simulink model "Bebop_sim_joystick_pathtrack"  (R2018a)
settings: Solver=VariableStepAuto  StartTime=0.0  StopTime=50  FixedStep=.05  MaxStep=0.3  MinStep=0.002
values from neighbouring files (symbols this model uses):
  g = 9.81    [initialize_race_no_realtime.m]    (also in initialize_race_realtime.m; initialize_race_realtime_backup_cubic.m; moving_average_rls_own.m = P(i-1)*meas*(lambda+meas*P(i-1)*meas)^-1)
  max_theta_X = (40)*pi/180    (= 0.698131700798)    [Bebop_sim_init.m]    (also in initialize_race_no_realtime.m = 0.13962634016; initialize_race_realtime.m = 1.308996939; initialize_race_realtime_backup_cubic.m = 1.308996939; run_batch1.m = list_agility(idx_agility)*max_theta_X)
  max_theta_Y = (40)*pi/180    (= 0.698131700798)    [Bebop_sim_init.m]    (also in initialize_race_no_realtime.m = 0.13962634016; initialize_race_realtime.m = 1.308996939; initialize_race_realtime_backup_cubic.m = 1.308996939; run_batch1.m = list_agility(idx_agility)*max_theta_Y)
  max_v_Z = .5    (= 0.5)    [Bebop_sim_init.m]    (also in initialize_race_no_realtime.m = 1; initialize_race_realtime.m = 3; initialize_race_realtime_backup_cubic.m = 3; run_batch1.m = list_agility(idx_agility)*max_v_Z)
libraries: simulink x2, sharedtransform x1, vrlib x1
settings Model: EnablePacing=on  Creator=vinni  LastModifiedBy=vinni
settings HardwareCC: ProdBitPerLong=64  ProdHWDeviceType=Intel->x86-64 (Linux 64)

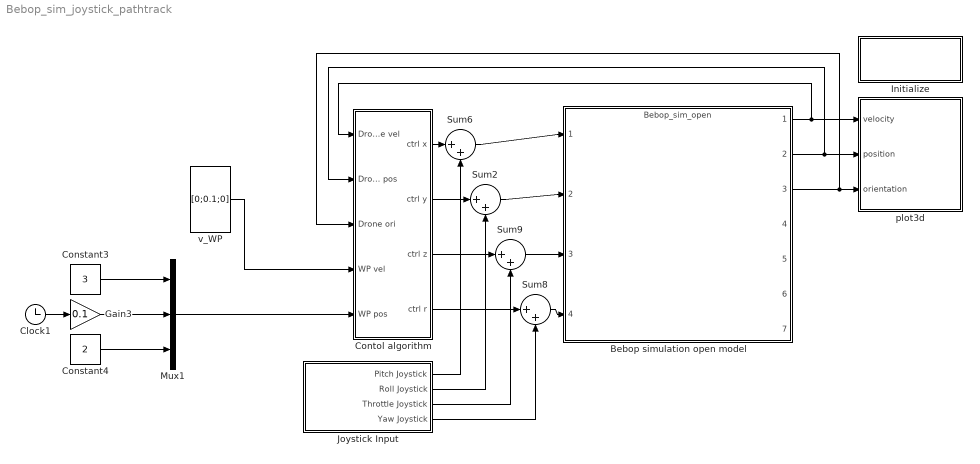
== system Bebop_sim_joystick_pathtrack ==
  Bebop simulation open model : ModelReference  ModelNameDialog=Bebop_sim_open.slx  SimulationMode=Normal  ModelReferenceVersion=1.31
  Clock1 : Clock
  Constant3 : Constant  Value=3
  Constant4 : Constant  Value=2
  Contol algorithm : Subsystem
  Gain3 : Gain  Gain=0.1
  Initialize : Subsystem  TreatAsAtomicUnit=on
  Joystick Input : Subsystem
  Mux1 : Mux  Inputs=3
  Sum{2,6,8..9} (4 alike) : Sum  Inputs=|++
  plot3d : MATLAB Function  TreatAsAtomicUnit=on
  v_WP : Constant  Value=[0;0.1;0]  VectorParams1D=off
  wires:
  Bebop simulation open model/2 -> plot3d/2(position), Contol algorithm/2(Drone pos)
  Bebop simulation open model/3 -> plot3d/3(orientation), Contol algorithm/3(Drone ori)
  Sum2/1 -> Bebop simulation open model/2
  Joystick Input/2(Roll Joystick) -> Sum2/2
  Joystick Input/1(Pitch Joystick) -> Sum6/2
  Joystick Input/4(Yaw Joystick) -> Sum8/2
  Joystick Input/3(Throttle Joystick) -> Sum9/2
  Bebop simulation open model/1 -> Contol algorithm/1(Drone vel), plot3d/1(velocity)
  Sum6/1 -> Bebop simulation open model/1
  Sum8/1 -> Bebop simulation open model/4
  Clock1/1 -> Gain3/1
  Sum9/1 -> Bebop simulation open model/3
  Gain3/1 -> Mux1/2
  Constant3/1 -> Mux1/1
  Constant4/1 -> Mux1/3
  v_WP/1 -> Contol algorithm/4(WP vel)
  Mux1/1 -> Contol algorithm/5(WP pos)
  Contol algorithm/1(ctrl x) -> Sum6/1
  Contol algorithm/2(ctrl y) -> Sum2/1
  Contol algorithm/3(ctrl z) -> Sum9/1
  Contol algorithm/4(ctrl r) -> Sum8/1

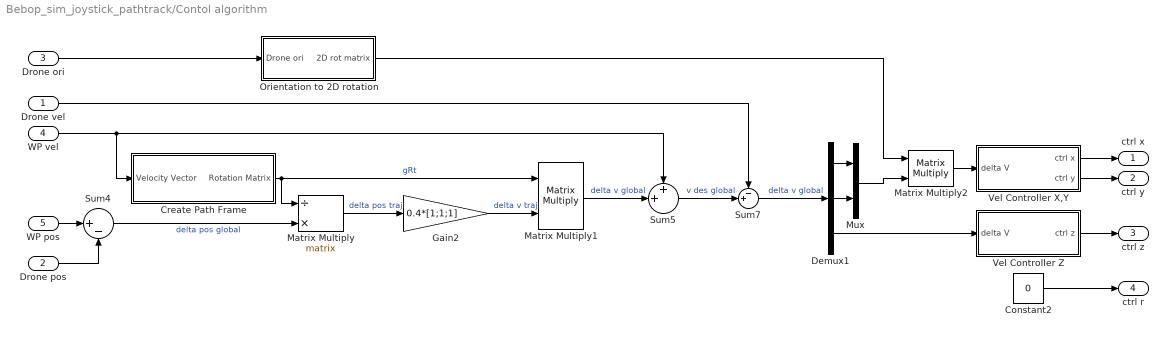
== system Bebop_sim_joystick_pathtrack/Contol algorithm ==
  Drone vel : Inport
  Drone pos : Inport  Port=2
  Drone ori : Inport  Port=3
  WP vel : Inport  Port=4
  WP pos : Inport  Port=5
  Constant2 : Constant  Value=0
  Create Path Frame : Subsystem
  Demux1 : Demux  Outputs=3
  Gain2 : Gain  Gain=0.4*[1;1;1]
  Matrix Multiply : Product  Inputs=/*  Multiplication=Matrix(*)
  Matrix Multiply1 : Product  Inputs=**  Multiplication=Matrix(*)
  Matrix Multiply2 : Product  Inputs=**  Multiplication=Matrix(*)
  Mux : Mux  Inputs=2
  Orientation to 2D rotation : Subsystem
  Sum4 : Sum  Inputs=|+-
  Sum5 : Sum  Inputs=++|
  Sum7 : Sum  Inputs=-+|
  Vel Controller X,Y : Subsystem
  Vel Controller Z : Subsystem
  ctrl x : Outport
  ctrl y : Outport  Port=2
  ctrl z : Outport  Port=3
  ctrl r : Outport  Port=4
  wires:
  Demux1/1 -> Mux/1
  Sum4/1 -> Matrix Multiply/2  "delta pos global"
  Matrix Multiply/1 -> Gain2/1  "delta pos traj"
  Mux/1 -> Matrix Multiply2/2
  Create Path Frame/1(Rotation Matrix) -> Matrix Multiply/1, Matrix Multiply1/1  "gRt"
  Constant2/1 -> ctrl r/1
  Demux1/2 -> Mux/2
  WP vel/1 -> Create Path Frame/1(Velocity Vector), Sum5/1
  Drone pos/1 -> Sum4/2
  Matrix Multiply2/1 -> Vel Controller X,Y/1(delta V)
  WP pos/1 -> Sum4/1
  Drone vel/1 -> Sum7/1
  Matrix Multiply1/1 -> Sum5/2  "delta v global"
  Vel Controller X,Y/2(ctrl y) -> ctrl y/1
  Sum7/1 -> Demux1/1  "delta v global"
  Vel Controller X,Y/1(ctrl x) -> ctrl x/1
  Sum5/1 -> Sum7/2  "v des global"
  Demux1/3 -> Vel Controller Z/1(delta V)
  Vel Controller Z/1(ctrl z) -> ctrl z/1
  Gain2/1 -> Matrix Multiply1/2  "delta v traj"
  Drone ori/1 -> Orientation to 2D rotation/1(Drone ori)
  Orientation to 2D rotation/1(2D rot matrix) -> Matrix Multiply2/1

== system Bebop_sim_joystick_pathtrack/Initialize ==
  Event Listener : EventListener  DisableCoverage=on  EventName=reset
  reset_plot : MATLAB Function  TreatAsAtomicUnit=on

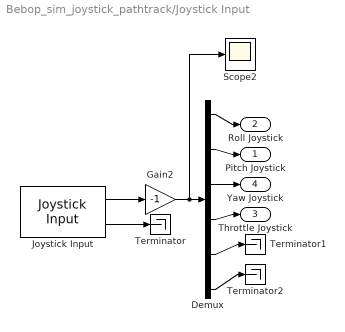
== system Bebop_sim_joystick_pathtrack/Joystick Input ==
  Demux : Demux  Outputs=6
  Gain2 : Gain  Gain=-1
  Joystick Input : vrlib/Joystick Input  joyid=1  adjustports=on  forcefeed=on
      settings: SourceProductBaseCode=VR
  Scope2 : Scope
  Terminator : Terminator
  Terminator1 : Terminator
  Terminator2 : Terminator
  Pitch Joystick : Outport
  Roll Joystick : Outport  Port=2
  Throttle Joystick : Outport  Port=3
  Yaw Joystick : Outport  Port=4
  wires:
  Demux/6 -> Terminator2/1
  Demux/5 -> Terminator1/1
  Demux/2 -> Pitch Joystick/1
  Joystick Input/1 -> Gain2/1
  Demux/1 -> Roll Joystick/1
  Demux/3 -> Yaw Joystick/1
  Gain2/1 -> Scope2/1, Demux/1
  Demux/4 -> Throttle Joystick/1
  Joystick Input/2 -> Terminator/1

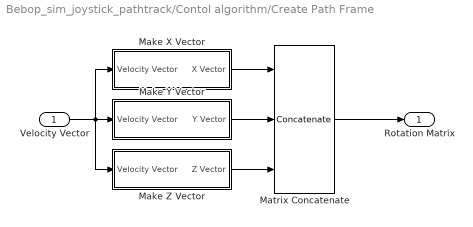
== system Bebop_sim_joystick_pathtrack/Contol algorithm/Create Path Frame ==
  Velocity Vector : Inport
  Make X Vector : Subsystem
  Make Y Vector : Subsystem
  Make Z Vector : Subsystem
  Matrix Concatenate : Concatenate  NumInputs=3  Mode=Multidimensional array  ConcatenateDimension=2
  Rotation Matrix : Outport
  wires:
  Velocity Vector/1 -> Make Z Vector/1(Velocity Vector), Make X Vector/1(Velocity Vector), Make Y Vector/1(Velocity Vector)
  Make Y Vector/1(Y Vector) -> Matrix Concatenate/2
  Make X Vector/1(X Vector) -> Matrix Concatenate/1
  Make Z Vector/1(Z Vector) -> Matrix Concatenate/3
  Matrix Concatenate/1 -> Rotation Matrix/1

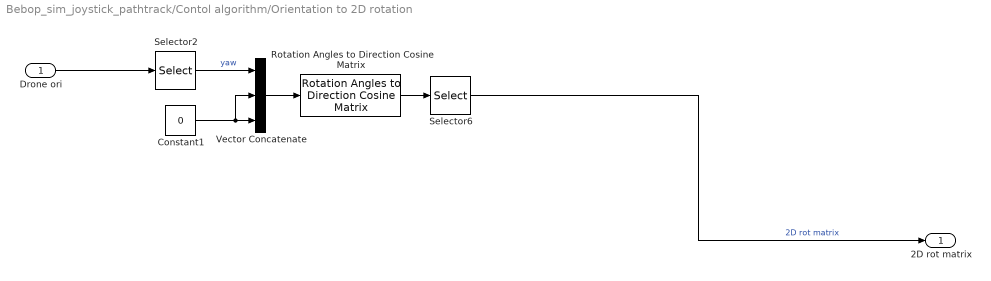
== system Bebop_sim_joystick_pathtrack/Contol algorithm/Orientation to 2D rotation ==
  Drone ori : Inport
  Constant1 : Constant  Value=0
  Rotation Angles to Direction Cosine Matrix : sharedtransform/Rotation Angles to Direction Cosine Matrix  rotationOrder=ZYX  aMode=aMode
      settings: SourceProductBaseCode=AE
  Selector2 : Selector  InputPortWidth=3  IndexOptions=Index vector (dialog)  Indices=3  OutputSizes=1
  Selector6 : Selector  NumberOfDimensions=2  InputPortWidth=3  IndexOptions=Index vector (dialog),Index vector (dialog)  Indices=[1,2],[1,2]  OutputSizes=1,1
  Vector Concatenate : Concatenate  NumInputs=3
  2D rot matrix : Outport
  wires:
  Constant1/1 -> Vector Concatenate/2, Vector Concatenate/3
  Rotation Angles to Direction Cosine Matrix/1 -> Selector6/1
  Vector Concatenate/1 -> Rotation Angles to Direction Cosine Matrix/1
  Selector2/1 -> Vector Concatenate/1  "yaw"
  Selector6/1 -> 2D rot matrix/1  "2D rot matrix"
  Drone ori/1 -> Selector2/1

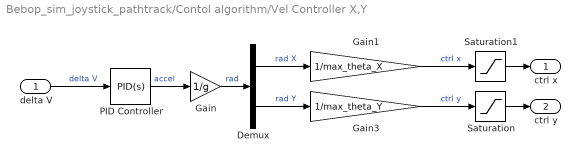
== system Bebop_sim_joystick_pathtrack/Contol algorithm/Vel Controller X,Y ==
  delta V : Inport
  Demux : Demux  Outputs=2
  Gain : Gain  Gain=1/g
  Gain1 : Gain  Gain=1/max_theta_X
  Gain3 : Gain  Gain=1/max_theta_Y
  PID Controller : simulink/Continuous/PID Controller  Controller=PID  TimeDomain=Continuous-time  SampleTime=-1  IntegratorMethod=Forward Euler  FilterMethod=Forward Euler  Form=Parallel  UseFilter=on  ControllerParametersSource=internal  P=0.7  I=0  D=0.01  N=10  InitialConditionSource=internal  InitialConditionForIntegrator=0  InitialConditionForFilter=0  ExternalReset=none  LimitOutput=off  UpperSaturationLimit=inf  LowerSaturationLimit=-inf  LinearizeAsGain=on  AntiWindupMode=none  Kb=1  TrackingMode=off  Kt=1  PParamMin=[]  PParamMax=[]  IParamMin=[]  IParamMax=[]  DParamMin=[]  DParamMax=[]  NParamMin=[]  NParamMax=[]  KbParamMin=[]  KbParamMax=[]  KtParamMin=[]  KtParamMax=[]  POutMin=[]  POutMax=[]  IOutMin=[]  IOutMax=[]  DOutMin=[]  DOutMax=[]  NOutMin=[]  NOutMax=[]  KbOutMin=[]  KbOutMax=[]  KtOutMin=[]  KtOutMax=[]  IntegratorOutMin=[]  IntegratorOutMax=[]  FilterOutMin=[]  FilterOutMax=[]  SumOutMin=[]  SumOutMax=[]  SumI1OutMin=[]  SumI1OutMax=[]  SumI2OutMin=[]  SumI2OutMax=[]  SumI3OutMin=[]  SumI3OutMax=[]  SumDOutMin=[]  SumDOutMax=[]  SaturationOutMin=[]  SaturationOutMax=[]  IntegratorContinuousStateAttributes=''  IntegratorStateMustResolveToSignalObject=off  IntegratorRTWStateStorageClass=Auto  FilterContinuousStateAttributes=''  FilterStateMustResolveToSignalObject=off  FilterRTWStateStorageClass=Auto  DifferentiatorICPrevScaledInput=0  DifferentiatorOutMin=[]  DifferentiatorOutMax=[]  FilterDiffOutCoefMin=[]  FilterDiffOutCoefMax=[]  SumDenOutMin=[]  SumDenOutMax=[]  SumNumOutMin=[]  SumNumOutMax=[]  ReciprocalOutMin=[]  ReciprocalOutMax=[]  DivideOutMin=[]  DivideOutMax=[]  TunerSelectOption=Transfer Function Based (PID Tuner App)
  Saturation : Saturate  UpperLimit=1  LowerLimit=-1
  Saturation1 : Saturate  UpperLimit=1  LowerLimit=-1
  ctrl x : Outport
  ctrl y : Outport  Port=2
  wires:
  delta V/1 -> PID Controller/1  "delta V"
  PID Controller/1 -> Gain/1  "accel"
  Gain1/1 -> Saturation1/1  "ctrl x"
  Demux/2 -> Gain3/1  "rad Y"
  Gain3/1 -> Saturation/1  "ctrl y"
  Gain/1 -> Demux/1  "rad"
  Demux/1 -> Gain1/1  "rad X"
  Saturation1/1 -> ctrl x/1
  Saturation/1 -> ctrl y/1

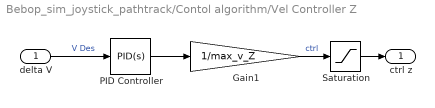
== system Bebop_sim_joystick_pathtrack/Contol algorithm/Vel Controller Z ==
  delta V : Inport
  Gain1 : Gain  Gain=1/max_v_Z
  PID Controller : simulink/Continuous/PID Controller  Controller=PID  TimeDomain=Continuous-time  SampleTime=-1  IntegratorMethod=Forward Euler  FilterMethod=Forward Euler  Form=Parallel  UseFilter=on  ControllerParametersSource=internal  P=10  I=2  D=0.01  N=10  InitialConditionSource=internal  InitialConditionForIntegrator=0  InitialConditionForFilter=0  ExternalReset=none  LimitOutput=off  UpperSaturationLimit=inf  LowerSaturationLimit=-inf  LinearizeAsGain=on  AntiWindupMode=none  Kb=1  TrackingMode=off  Kt=1  PParamMin=[]  PParamMax=[]  IParamMin=[]  IParamMax=[]  DParamMin=[]  DParamMax=[]  NParamMin=[]  NParamMax=[]  KbParamMin=[]  KbParamMax=[]  KtParamMin=[]  KtParamMax=[]  POutMin=[]  POutMax=[]  IOutMin=[]  IOutMax=[]  DOutMin=[]  DOutMax=[]  NOutMin=[]  NOutMax=[]  KbOutMin=[]  KbOutMax=[]  KtOutMin=[]  KtOutMax=[]  IntegratorOutMin=[]  IntegratorOutMax=[]  FilterOutMin=[]  FilterOutMax=[]  SumOutMin=[]  SumOutMax=[]  SumI1OutMin=[]  SumI1OutMax=[]  SumI2OutMin=[]  SumI2OutMax=[]  SumI3OutMin=[]  SumI3OutMax=[]  SumDOutMin=[]  SumDOutMax=[]  SaturationOutMin=[]  SaturationOutMax=[]  IntegratorContinuousStateAttributes=''  IntegratorStateMustResolveToSignalObject=off  IntegratorRTWStateStorageClass=Auto  FilterContinuousStateAttributes=''  FilterStateMustResolveToSignalObject=off  FilterRTWStateStorageClass=Auto  DifferentiatorICPrevScaledInput=0  DifferentiatorOutMin=[]  DifferentiatorOutMax=[]  FilterDiffOutCoefMin=[]  FilterDiffOutCoefMax=[]  SumDenOutMin=[]  SumDenOutMax=[]  SumNumOutMin=[]  SumNumOutMax=[]  ReciprocalOutMin=[]  ReciprocalOutMax=[]  DivideOutMin=[]  DivideOutMax=[]  TunerSelectOption=Transfer Function Based (PID Tuner App)
  Saturation : Saturate  UpperLimit=1  LowerLimit=-1
  ctrl z : Outport
  wires:
  Gain1/1 -> Saturation/1  "ctrl"
  delta V/1 -> PID Controller/1  "V Des"
  Saturation/1 -> ctrl z/1
  PID Controller/1 -> Gain1/1

== system Bebop_sim_joystick_pathtrack/Contol algorithm/Create Path Frame/Make X Vector ==
  Velocity Vector : Inport
  Make Unit : Subsystem
  X Vector : Outport
  wires:
  Velocity Vector/1 -> Make Unit/1(Vector)
  Make Unit/1(Unit Vector) -> X Vector/1

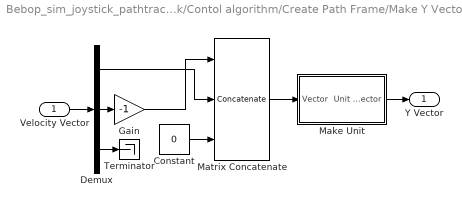
== system Bebop_sim_joystick_pathtrack/Contol algorithm/Create Path Frame/Make Y Vector ==
  Velocity Vector : Inport
  Constant : Constant  Value=0
  Demux : Demux  Outputs=3
  Gain : Gain  Gain=-1
  Make Unit : Subsystem
  Matrix Concatenate : Concatenate  NumInputs=3  Mode=Multidimensional array
  Terminator : Terminator
  Y Vector : Outport
  wires:
  Make Unit/1(Unit Vector) -> Y Vector/1
  Velocity Vector/1 -> Demux/1
  Demux/3 -> Terminator/1
  Demux/2 -> Gain/1
  Gain/1 -> Matrix Concatenate/1
  Demux/1 -> Matrix Concatenate/2
  Constant/1 -> Matrix Concatenate/3
  Matrix Concatenate/1 -> Make Unit/1(Vector)

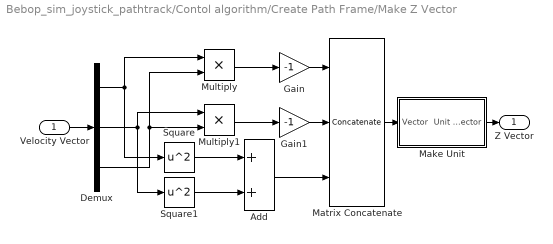
== system Bebop_sim_joystick_pathtrack/Contol algorithm/Create Path Frame/Make Z Vector ==
  Velocity Vector : Inport
  Add : Sum
  Demux : Demux  Outputs=3
  Gain : Gain  Gain=-1
  Gain1 : Gain  Gain=-1
  Make Unit : Subsystem
  Matrix Concatenate : Concatenate  NumInputs=3  Mode=Multidimensional array
  Multiply : Product
  Multiply1 : Product
  Square : Math  Operator=square  SaturateOnIntegerOverflow=on
  Square1 : Math  Operator=square  SaturateOnIntegerOverflow=on
  Z Vector : Outport
  wires:
  Make Unit/1(Unit Vector) -> Z Vector/1
  Velocity Vector/1 -> Demux/1
  Demux/3 -> Multiply/2, Multiply1/2
  Matrix Concatenate/1 -> Make Unit/1(Vector)
  Multiply/1 -> Gain/1
  Gain/1 -> Matrix Concatenate/1
  Demux/1 -> Square/1, Multiply/1
  Multiply1/1 -> Gain1/1
  Gain1/1 -> Matrix Concatenate/2
  Demux/2 -> Square1/1, Multiply1/1
  Add/1 -> Matrix Concatenate/3
  Square/1 -> Add/1
  Square1/1 -> Add/2

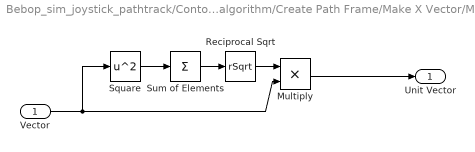
== system Bebop_sim_joystick_pathtrack/Contol algorithm/Create Path Frame/Make X Vector/Make Unit ==
  Vector : Inport
  Multiply : Product
  Reciprocal Sqrt : Sqrt  Operator=rSqrt  SaturateOnIntegerOverflow=on
  Square : Math  Operator=square  SaturateOnIntegerOverflow=on
  Sum of Elements : Sum  Inputs=+
  Unit Vector : Outport
  wires:
  Reciprocal Sqrt/1 -> Multiply/1
  Vector/1 -> Square/1, Multiply/2
  Square/1 -> Sum of Elements/1
  Multiply/1 -> Unit Vector/1
  Sum of Elements/1 -> Reciprocal Sqrt/1

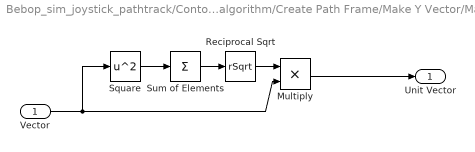
== system Bebop_sim_joystick_pathtrack/Contol algorithm/Create Path Frame/Make Y Vector/Make Unit ==
  Vector : Inport
  Multiply : Product
  Reciprocal Sqrt : Sqrt  Operator=rSqrt  SaturateOnIntegerOverflow=on
  Square : Math  Operator=square  SaturateOnIntegerOverflow=on
  Sum of Elements : Sum  Inputs=+
  Unit Vector : Outport
  wires:
  Reciprocal Sqrt/1 -> Multiply/1
  Vector/1 -> Square/1, Multiply/2
  Square/1 -> Sum of Elements/1
  Multiply/1 -> Unit Vector/1
  Sum of Elements/1 -> Reciprocal Sqrt/1

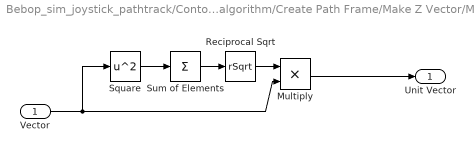
== system Bebop_sim_joystick_pathtrack/Contol algorithm/Create Path Frame/Make Z Vector/Make Unit ==
  Vector : Inport
  Multiply : Product
  Reciprocal Sqrt : Sqrt  Operator=rSqrt  SaturateOnIntegerOverflow=on
  Square : Math  Operator=square  SaturateOnIntegerOverflow=on
  Sum of Elements : Sum  Inputs=+
  Unit Vector : Outport
  wires:
  Reciprocal Sqrt/1 -> Multiply/1
  Vector/1 -> Square/1, Multiply/2
  Square/1 -> Sum of Elements/1
  Multiply/1 -> Unit Vector/1
  Sum of Elements/1 -> Reciprocal Sqrt/1

== matlab function Bebop_sim_joystick_pathtrack/plot3d ==
  data: velocity input; position input; orientation input
function plot3d(velocity, position, orientation)
coder.extrinsic('delete')

children = get(gca, 'children');
delete(children(1:4));

% for id=1:5
%     v = 0;
%     v = get(children(id),'MarkerSize');
%     if v == 6
%         delete(children(id));
%     end
% end




gRb = eul2rotm([orientation(3),orientation(2),orientation(1)]);
length = 0.3;
x_bebop = gRb*[length;0;0];
y_bebop = gRb*[0;length;0];
z_bebop = gRb*[0;0;length];


plot3(position(1),position(2),position(3),'m.','MarkerSize',7)
plot3(position(1),position(2),0,'k.','MarkerSize',5)

plot3(position(1)+[0 velocity(1)],position(2)+[0 velocity(2)],position(3)+[0 velocity(3)],'k-','LineWidth',2)

plot3(position(1)+[0 x_bebop(1)],position(2)+[0 x_bebop(2)],position(3)+[0 x_bebop(3)],'r-')
plot3(position(1)+[0 y_bebop(1)],position(2)+[0 y_bebop(2)],position(3)+[0 y_bebop(3)],'g-')
plot3(position(1)+[0 z_bebop(1)],position(2)+[0 z_bebop(2)],position(3)+[0 z_bebop(3)],'b-')

== matlab function Bebop_sim_joystick_pathtrack/Initialize/reset_plot ==
function reset_plot()
close all;
figure('units','normalized','outerposition',[0 0 0.5 1])
hold on
grid on
axis equal
plot3(0,0,0,'m.')
plot3(0,0,0,'m.')
plot3(0,0,0,'m.')
plot3(0,0,0,'m.')
% axis([-5,5,-5,5,-2,2])
axis([-1,10,-5,5,0,4])
%view(-20,40) % 3D view
%view(-90,90) % top view
view(-90,0) % front view
xlabel('x')
ylabel('y')
zlabel('z')
